simulink model "bike_lane_keeper_mpc"  (R2025b)
settings: Solver=FixedStepAuto  StartTime=0.0  StopTime=10.0  FixedStep=dt  RelTol=1e-3
values from neighbouring files (symbols this model uses):
  dt = 0.05    [simulink_init.m]
  H = [1, 0, 0, 0 ... (first row only)    [simulink_init.m]
  max_turn = deg2rad(25)    [simulink_init.m]
  P_hat_0 = diag([5, 5, 5, 5])    [simulink_init.m]
  Q_kf = diag([1e-3, 1e-2, 4e-3, 2e-3])    [simulink_init.m]
  Q_mpc = diag([30, 1, 40, 5])    [simulink_init.m]
  R_kf = diag([0.08.^2, deg2rad(1.5).^2])    [simulink_init.m]
  R_mpc = 100    [simulink_init.m]
  x_0 = [-0.7; 0.2; deg2rad(4); -0.1]    [simulink_init.m]
  x_hat_0 = [1; 0; deg2rad(0.5); 0]    [simulink_init.m]
undefined symbols (not defined in the file or in its folder): Ad, Bd, Cd, Dd, Ed, F, Gamma, Phi
libraries: simulink x2
settings Model: Creator=benstarkey  LastModifiedBy=benstarkey
settings OptimizationCC: DefaultParameterBehavior=Inlined  EnhancedBackFolding=on  PassReuseOutputArgsAs=Individual arguments  ZeroExternalMemoryAtStartup=off  ZeroInternalMemoryAtStartup=off  OptimizeBlockOrder=speed  DifferentSizesBufferReuse=on  OptimizationCustomize=off  EfficientTunableParamExpr=on
settings DebuggingCC: ParameterTunabilityLossMsg=error
settings SFSimCC: MATLABDynamicMemAlloc=off
settings RTWCC: SystemTargetFile=ert.tlc  GenCodeOnly=on  TemplateMakefile=ert_default_tmf  TargetLang=C++  Description=Embedded Coder
settings CodeAppCC: ForceParamTrailComments=on  IgnoreCustomStorageClasses=off  OperatorAnnotations=on  SimulinkDataObjDesc=on  SFDataObjDesc=on  InsertBlockDesc=on
settings ERTTargetCC: RootIOFormat=Structure reference  ERTCustomFileTemplate=example_file_process.tlc  TargetLangStandard=C++11 (ISO)  GenerateSampleERTMain=on  CodeInterfacePackaging=C++ class  SubcomponentCodeInterfacePackaging=C++ class

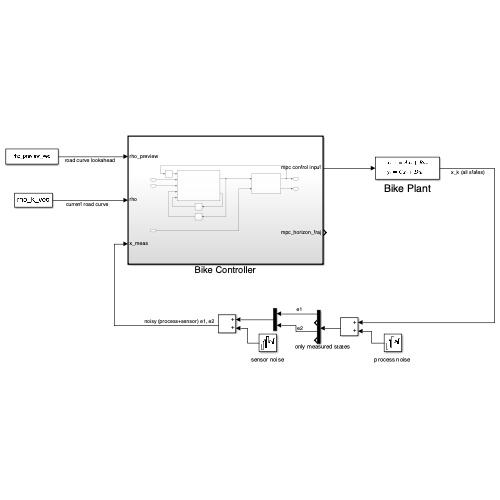
[thumbnail: Simulink's stored preview of the top-level diagram]
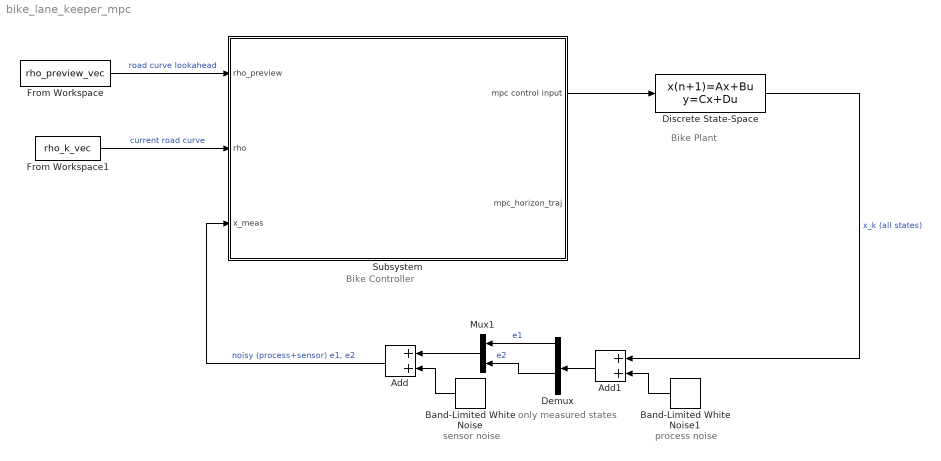
== system bike_lane_keeper_mpc ==
  note: Bike Controller
  note: only measured states
  note: sensor noise
  note: process noise
  note: Bike Plant
  Add : Sum
  Add1 : Sum
  Band-Limited White Noise : simulink/Sources/Band-Limited White Noise  Cov=sensor_noise_power  Ts=dt  seed=[23341]
  Band-Limited White Noise1 : simulink/Sources/Band-Limited White Noise  Cov=process_noise_power  Ts=dt  seed=[23341]
  Demux : Demux
  Discrete State-Space : DiscreteStateSpace  A=Ad  B=[Bd, Ed]  C=Cd  D=Dd  InitialCondition=x_0  SampleTime=dt
  From Workspace : FromWorkspace  VariableName=rho_preview_vec  SampleTime=dt  OutputAfterFinalValue=Holding final value
  From Workspace1 : FromWorkspace  VariableName=rho_k_vec  SampleTime=dt  OutputAfterFinalValue=Holding final value
  Mux1 : Mux  Inputs=2
  Subsystem : Subsystem  TreatAsAtomicUnit=on  SystemSampleTime=dt
      settings: MinAlgLoopOccurrences=on
  wires:
  Subsystem/1(mpc control input) -> Discrete State-Space/1
  Discrete State-Space/1 -> Add1/1  "x_k (all states)"
  Demux/1 -> Mux1/1  "e1"
  Demux/3 -> Mux1/2  "e2"
  Add/1 -> Subsystem/3(x_meas)  "noisy (process+sensor) e1, e2"
  Add1/1 -> Demux/1
  Band-Limited White Noise1/1 -> Add1/2
  Band-Limited White Noise/1 -> Add/2
  Mux1/1 -> Add/1
  From Workspace1/1 -> Subsystem/2(rho)  "current road curve"
  From Workspace/1 -> Subsystem/1(rho_preview)  "road curve lookahead"

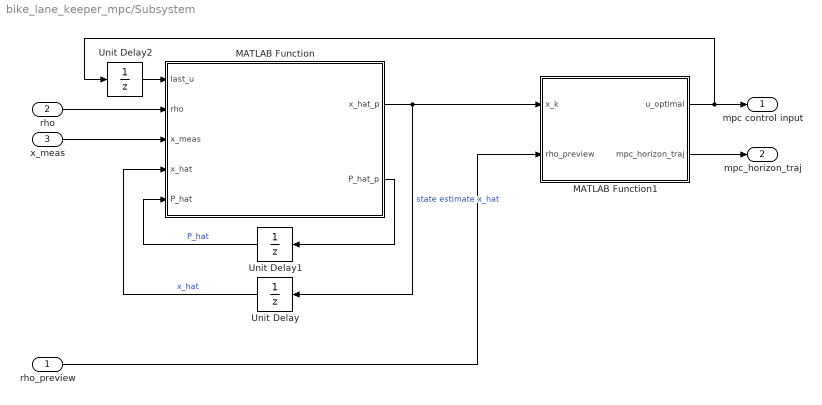
== system bike_lane_keeper_mpc/Subsystem ==
  rho_preview : Inport
  rho : Inport  Port=2
  x_meas : Inport  Port=3
  MATLAB Function : MATLAB Function  TreatAsAtomicUnit=on  mask{Ad=Ad, Bd=Bd, Ed=Ed, H=H, Q_kf=Q_kf, R_kf=R_kf}
      mask prompts: Ad "Dynamic Matrix (Ad)"; Bd "Control Matrix (Bd)"; Ed "Disturbance Matrix (Ed)"; H "Kalman State Selection (H)"
  MATLAB Function1 : MATLAB Function  TreatAsAtomicUnit=on  mask{F=F, Phi=Phi, Gamma=Gamma, Q=Q_mpc, R=R_mpc, u_max=max_turn}
      mask prompts: F "State Horizon (F)"; Phi "Control Horizon (Phi)"; Gamma "Disturbance Horizon (Gamma)"; Q "State Cost (Q)"; R "Control Cost (R)"; u_max "Max Steering Angle"
  Unit Delay : UnitDelay  InitialCondition=x_hat_0  SampleTime=dt  HasFrameUpgradeWarning=on
  Unit Delay1 : UnitDelay  InitialCondition=P_hat_0  SampleTime=dt  HasFrameUpgradeWarning=on
  Unit Delay2 : UnitDelay  SampleTime=dt  HasFrameUpgradeWarning=on
  mpc control input : Outport
  mpc_horizon_traj : Outport  Port=2
  wires:
  x_meas/1 -> MATLAB Function/3(x_meas)
  MATLAB Function1/1(u_optimal) -> mpc control input/1, Unit Delay2/1
  MATLAB Function/1(x_hat_p) -> MATLAB Function1/1(x_k), Unit Delay/1  "state estimate x_hat"
  rho_preview/1 -> MATLAB Function1/2(rho_preview)
  MATLAB Function/2(P_hat_p) -> Unit Delay1/1
  Unit Delay1/1 -> MATLAB Function/5(P_hat)  "P_hat"
  Unit Delay2/1 -> MATLAB Function/1(last_u)
  MATLAB Function1/2(mpc_horizon_traj) -> mpc_horizon_traj/1
  rho/1 -> MATLAB Function/2(rho)
  Unit Delay/1 -> MATLAB Function/4(x_hat)  "x_hat"

== matlab function bike_lane_keeper_mpc/Subsystem/MATLAB Function1 ==
  data: x_k input; u_optimal output; rho_preview input; F parameter; Phi parameter; Gamma parameter; Q parameter; R parameter; u_max parameter; mpc_horizon_traj output
function [u_optimal, mpc_horizon_traj] = MPController(x_k, rho_preview, F, Phi, Gamma, Q, R, u_max)
%#codegen

% Define x_k as column vector [4x1]
x_k_col = x_k(:);

% Solve 
[u_optimal, u_horizon] = mpc_solve_active_set(x_k_col, F, Phi, Gamma, rho_preview, Q, R, u_max);

% Calculate mpc planned trajectory
mpc_horizon_traj = F*x_k_col + Phi*u_horizon + Gamma*rho_preview;

end

== matlab function bike_lane_keeper_mpc/Subsystem/MATLAB Function ==
  data: last_u input; rho input; x_meas input; x_hat input; P_hat input; x_hat_p output; P_hat_p output; Ad parameter; Bd parameter; Ed parameter; H parameter; Q_kf parameter; R_kf parameter
function [x_hat_p, P_hat_p] = bike_kf(last_u, rho, x_meas, x_hat, P_hat, Ad, Bd, Ed, H, Q_kf, R_kf)
%#codegen

% Run kalman filter function from mpc folder
[x_hat_p, P_hat_p, ~] = kalman_filter(x_hat, last_u, P_hat, rho, x_meas, Ad, Bd, Ed, H, Q_kf, R_kf);

end
